simulink model "vgammaRegler"  (R2017a)
settings: Solver=VariableStepAuto  StartTime=0.0  StopTime=10.0  RelTol=1e-3
undefined symbols (not defined in the file or in its folder): G_mot, R_Kipp_Roboter
settings Model: Creator=Timo  LastModifiedBy=Timo

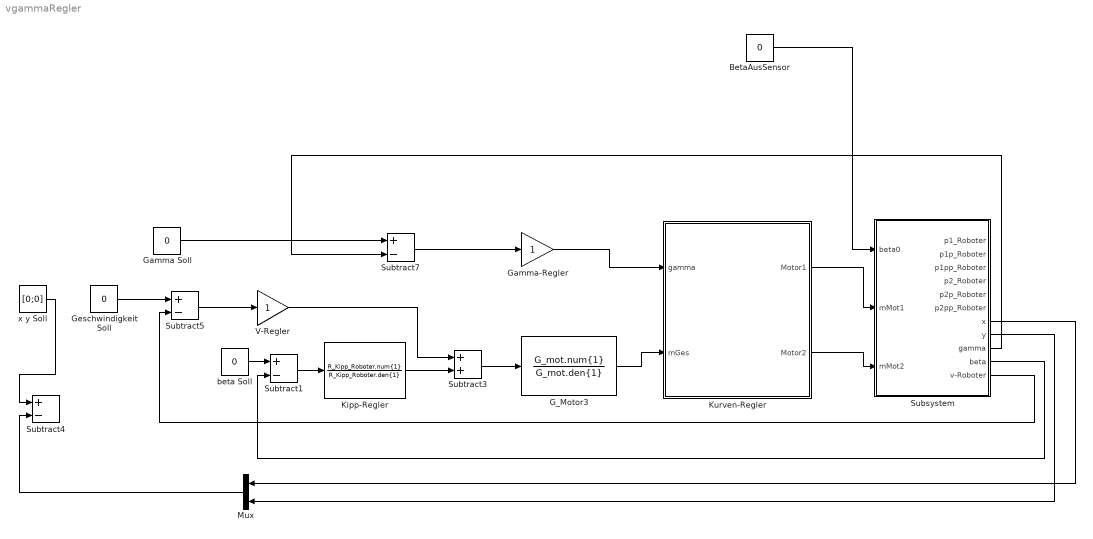
== system vgammaRegler ==
  BetaAusSensor : Constant  Value=0
  G_Motor3 : TransferFcn  Numerator=G_mot.num{1}  Denominator=G_mot.den{1}
  Gamma Soll : Constant  Value=0
  Gamma-Regler : Gain
  Geschwindigkeit Soll : Constant  Value=0
  Kipp-Regler : TransferFcn  Numerator=R_Kipp_Roboter.num{1}  Denominator=R_Kipp_Roboter.den{1}
  Kurven-Regler : Subsystem
  Mux : Mux  Inputs=2
  Subsystem : Subsystem
  Subtract{1,4..5,7} (4 alike) : Sum  Inputs=+-
  Subtract3 : Sum
  V-Regler : Gain
  beta Soll : Constant  Value=0
  x y Soll : Constant  Value=[0;0]
  wires:
  Subsystem/7(x) -> Mux/1
  Subsystem/8(y) -> Mux/2
  Mux/1 -> Subtract4/2
  x y Soll/1 -> Subtract4/1
  Kipp-Regler/1 -> Subtract3/2
  Subtract1/1 -> Kipp-Regler/1
  beta Soll/1 -> Subtract1/1
  Subsystem/10(beta) -> Subtract1/2
  V-Regler/1 -> Subtract3/1
  Kurven-Regler/2(Motor2) -> Subsystem/3(mMot2)
  Kurven-Regler/1(Motor1) -> Subsystem/2(mMot1)
  Subtract3/1 -> G_Motor3/1
  G_Motor3/1 -> Kurven-Regler/2(mGes)
  Subtract7/1 -> Gamma-Regler/1
  Geschwindigkeit Soll/1 -> Subtract5/1
  Subtract5/1 -> V-Regler/1
  Subsystem/11(v-Roboter) -> Subtract5/2
  BetaAusSensor/1 -> Subsystem/1(beta0)
  Subsystem/9(gamma) -> Subtract7/2
  Gamma-Regler/1 -> Kurven-Regler/1(gamma)
  Gamma Soll/1 -> Subtract7/1

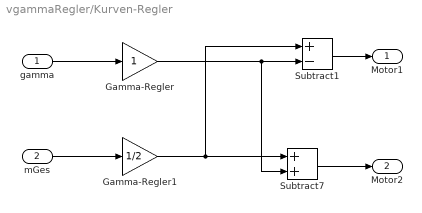
== system vgammaRegler/Kurven-Regler ==
  gamma : Inport
  mGes : Inport  Port=2
  Gamma-Regler : Gain
  Gamma-Regler1 : Gain  Gain=1/2
  Subtract1 : Sum  Inputs=+-
  Subtract7 : Sum
  Motor1 : Outport
  Motor2 : Outport  Port=2
  wires:
  gamma/1 -> Gamma-Regler/1
  mGes/1 -> Gamma-Regler1/1
  Gamma-Regler/1 -> Subtract1/2, Subtract7/2
  Subtract7/1 -> Motor2/1
  Subtract1/1 -> Motor1/1
  Gamma-Regler1/1 -> Subtract1/1, Subtract7/1

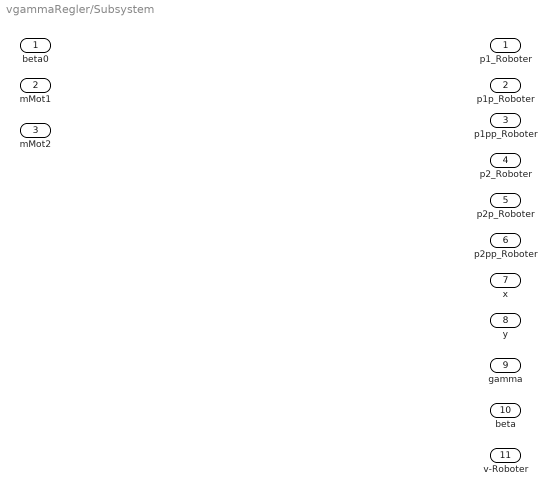
== system vgammaRegler/Subsystem ==
  beta0 : Inport
  mMot1 : Inport  Port=2
  mMot2 : Inport  Port=3
  p1_Roboter : Outport
  p1p_Roboter : Outport  Port=2
  p1pp_Roboter : Outport  Port=3
  p2_Roboter : Outport  Port=4
  p2p_Roboter : Outport  Port=5
  p2pp_Roboter : Outport  Port=6
  x : Outport  Port=7
  y : Outport  Port=8
  gamma : Outport  Port=9
  beta : Outport  Port=10
  v-Roboter : Outport  Port=11
